simulink model "CommandEnEffort"  (R2020b)
settings: Solver=FixedStepAuto  StartTime=0.0  StopTime=10  RelTol=1e-3
undefined symbols (not defined in the file): B, Beta, kc, ke, ki, kp, M, w0, wu, x
settings Model: Creator=Laura  LastModifiedBy=Laura

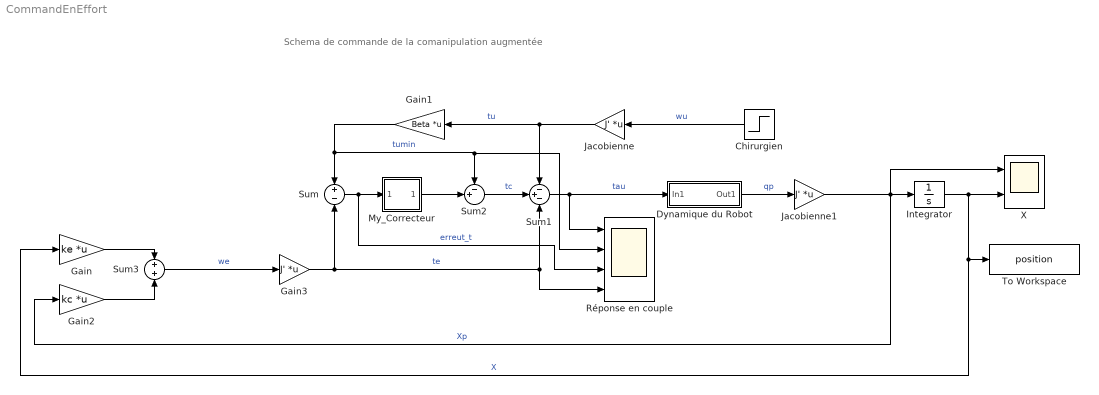
== system CommandEnEffort ==
  note: Schema de commande de la comanipulation augmentée
  Chirurgien : Step  Before=w0  After=wu  SampleTime=0  VectorParams1D=off
  Dynamique du Robot : Subsystem
      mask Display: disp('(Ms + B)^-1')
  Gain : Gain  Gain=ke  Multiplication=Matrix(K*u)
  Gain1 : Gain  Gain=Beta  Multiplication=Matrix(K*u)
  Gain2 : Gain  Gain=kc  Multiplication=Matrix(K*u)
  Gain3 : Gain  Gain=J'  Multiplication=Matrix(K*u)
  Integrator : Integrator  InitialCondition=x
  Jacobienne : Gain  Gain=J'  Multiplication=Matrix(K*u)
  Jacobienne1 : Gain  Gain=J'  Multiplication=Matrix(K*u)
  My_Correcteur : Subsystem
      mask Display: disp('PI')
  Réponse en couple : Scope  NumInputPorts=4
  Sum : Sum  Inputs=+|-
  Sum1 : Sum  Inputs=-+-
  Sum2 : Sum  Inputs=-+|
  Sum3 : Sum  Inputs=+|+
  To Workspace : ToWorkspace  VariableName=position  SampleTime=0.03
  X : Scope  NumInputPorts=2
  wires:
  Gain3/1 -> Sum/2, Réponse en couple/4, Sum1/3  "te"
  Dynamique du Robot/1(Out1) -> Jacobienne1/1  "qp"
  Chirurgien/1 -> Jacobienne/1  "wu"
  Gain1/1 -> Réponse en couple/2, Sum2/1, Sum/1  "tumin"
  Sum2/1 -> Sum1/2  "tc"
  Jacobienne1/1 -> X/1, Gain2/1, Integrator/1  "Xp"
  Sum/1 -> Réponse en couple/3, My_Correcteur/1(erreut_t)  "erreut_t"
  My_Correcteur/1(Out1) -> Sum2/2
  Integrator/1 -> Gain/1, To Workspace/1, X/2  "X"
  Sum1/1 -> Réponse en couple/1, Dynamique du Robot/1(In1)  "tau"
  Gain/1 -> Sum3/1
  Gain2/1 -> Sum3/2
  Sum3/1 -> Gain3/1  "we"
  Jacobienne/1 -> Sum1/1, Gain1/1  "tu"

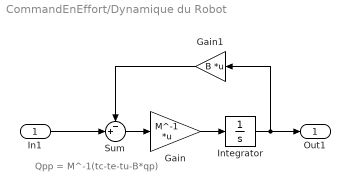
== system CommandEnEffort/Dynamique du Robot ==
  note: Qpp = M^-1(tc-te-tu-B*qp)
  In1 : Inport
  Gain : Gain  Gain=M^-1  Multiplication=Matrix(K*u)
  Gain1 : Gain  Gain=B  Multiplication=Matrix(K*u)
  Integrator : Integrator
  Sum : Sum  Inputs=-+|
  Out1 : Outport
  wires:
  Gain/1 -> Integrator/1
  Sum/1 -> Gain/1
  Gain1/1 -> Sum/1
  Integrator/1 -> Gain1/1, Out1/1
  In1/1 -> Sum/2

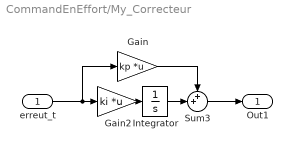
== system CommandEnEffort/My_Correcteur ==
  erreut_t : Inport
  Gain : Gain  Gain=kp  Multiplication=Matrix(K*u)
  Gain2 : Gain  Gain=ki  Multiplication=Matrix(K*u)
  Integrator : Integrator  InitialCondition=w0
  Sum3 : Sum  Inputs=++|
  Out1 : Outport
  wires:
  Sum3/1 -> Out1/1
  Gain/1 -> Sum3/1
  Gain2/1 -> Integrator/1
  Integrator/1 -> Sum3/2
  erreut_t/1 -> Gain/1, Gain2/1
